simulink model "gm_sampleModel71194_pp_7_1_sub"  (R2023b)
settings: Solver=VariableStepAuto  StartTime=0.0  StopTime=10.0  RelTol=1e-3
libraries: simulink x45, hdlsllib x1, hdlmdlgenlib x1
(part 1 of 2)
settings Model: Creator=CW  LastModifiedBy=CW
settings OptimizationCC: BlockReduction=off  ConditionallyExecuteInputs=off
settings DebuggingCC: ArtificialAlgebraicLoopMsg=none  InheritedTsInSrcMsg=none

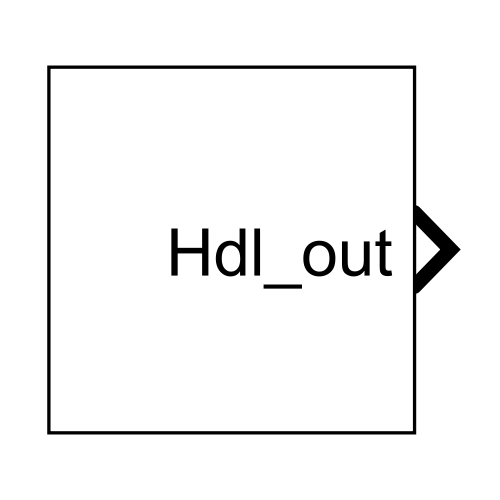
[thumbnail: Simulink's stored preview of the top-level diagram]
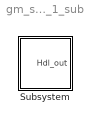
== system gm_sampleModel71194_pp_7_1_sub ==
  Subsystem : Subsystem

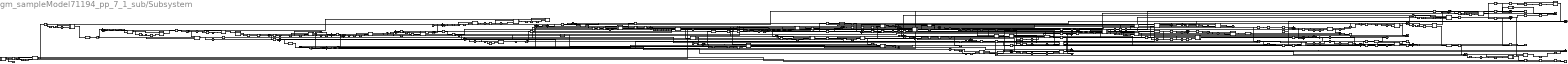
== system gm_sampleModel71194_pp_7_1_sub/Subsystem ==
  Reshape : Reshape
  Reshape1 : Reshape
  cfblk1 : Subsystem
  cfblk10 : Subsystem  mask(Compare To Zero){relop=<=, OutDataTypeStr=uint8, ZeroCross=on}
      mask prompts: relop "Simulink:masks:Operator_MP"; OutDataTypeStr "Simulink:masks:OutputDataType_MP"; ZeroCross "Simulink:masks:EnableZerocrossingDetection_MP"
      mask help: Simulink:masks:CompareToZero_MD
      mask init:
      | OutDataTypeStr = 'uint8';
      | ZeroCross = 'on';
      | blkName = 'sampleModel71194_pp_7_1_sub/Subsystem/cfblk10';
      | relop = '<=';
      | setValue = 'fixdt(0, 8)';
      mask TypeOptions relop: == | ~= | < | <= | >= | >
      mask TypeOptions OutDataTypeStr: Simulink:masks:uint8 | Simulink:masks:boolean
      mask Callback ZeroCross: sl('zeroCrossEnable', gcbh);
      mask Display: disp([relop,' 0'])
  cfblk100_inst : Subsystem
  cfblk{18,21,41,43,80..82,92,101,118,121,123} (12 alike) : Product  Inputs=*/  OutDataTypeStr=uint8  RndMeth=Zero  SaturateOnIntegerOverflow=on  SampleTime=1
  cfblk102_inst : Subsystem
  cfblk103 : Subsystem
  cfblk{20,22,29,33,36,40,64,72,77,88,90,94,104,111..112,115..116,125,128,141,143..144,152} (23 alike) : Sum  OutDataTypeStr=uint8  AccumDataTypeStr=uint8  SampleTime=1
  cfblk{49,58..59,74,105,108,110} (7 alike) : Signum  SampleTime=1
  cfblk{15,32,35,48,61,85,106,113,139..140} (10 alike) : MinMax  OutDataTypeStr=uint8
  cfblk{16,70,89,91,99,109,120,137,142,151} (10 alike) : Sum  Inputs=+-  OutDataTypeStr=uint8  AccumDataTypeStr=uint8  SampleTime=1
  cfblk11 : Subsystem
  cfblk{56,73,97,114,122} (5 alike) : ComplexToRealImag  SampleTime=1
  cfblk{34,53,69,71,86,96,98,117} (8 alike) : Sum  OutDataTypeStr=uint8  AccumDataTypeStr=uint8  RndMeth=Nearest  SampleTime=1
  cfblk117_const_val : Constant  Value=0  VectorParams1D=off  OutDataTypeStr=uint8  SampleTime=1
  cfblk119_inst : Subsystem
  cfblk12 : simulink/Logic and Bit Operations/Bit Set  iBit=double(0)
  cfblk124 : Subsystem  mask(Real World Value Increment){}
      mask help: Simulink:masks:RealWorldValueIncrement_MD
      mask Display: disp('V++')
  cfblk126_inst : Subsystem
  cfblk127 : Subsystem
  cfblk129 : Subsystem  mask(Real World Value Increment){}
      mask help: Simulink:masks:RealWorldValueIncrement_MD
      mask Display: disp('V++')
  cfblk13 : Subsystem  mask(Compare To Constant){relop=<=, const=double(3), OutDataTypeStr=uint8, ZeroCross=on}
      mask prompts: relop "Simulink:masks:Operator_MP"; const "Simulink:masks:ConstantValue_MP"; OutDataTypeStr "Simulink:masks:OutputDataType_MP"; ZeroCross "Simulink:masks:EnableZerocrossingDetection_MP"
      mask help: Simulink:masks:CompareToConstant_MD
      mask init:
      | OutDataTypeStr = 'uint8';
      | ZeroCross = 'on';
      | blkName = 'sampleModel71194_pp_7_1_sub/Subsystem/cfblk13';
      | const = double(3);
      | const_str = '3.0';
      | const_val = double(3);
      | relop = '<=';
      | setValue = 'fixdt(0, 8)';
      | str = '<= 3';
      mask TypeOptions relop: == | ~= | < | <= | >= | >
      mask TypeOptions OutDataTypeStr: Simulink:masks:uint8 | Simulink:masks:boolean
      mask Callback ZeroCross: sl('zeroCrossEnable', gcbh);
      mask Display: disp(str)
  cfblk130 : Subsystem
  cfblk131 : Subsystem
  cfblk{26,44,51,62,132,148} (6 alike) : Abs  SampleTime=1  OutDataTypeStr=uint8  SaturateOnIntegerOverflow=off
  cfblk133 : Subsystem
  cfblk134_inst : Subsystem
  cfblk135 : Subsystem
  cfblk136 : Subsystem
  cfblk{42,57,66,68,78..79,138,145..146} (9 alike) : Sum  Inputs=+  OutDataTypeStr=uint8
  cfblk14 : Subsystem  mask(Detect Fall Nonpositive){vinit=double(0), InputProcessing=Elements as channels (sample based), OutDataTypeStr=uint8}
      mask prompts: vinit "Simulink:masks:InitialCondition_MP"; InputProcessing "Simulink:masks:InputProcessing_MP"; OutDataTypeStr "Simulink:masks:OutputDataType_MP"
      mask help: Simulink:masks:DetectFallNonpositive_MD
      mask init:
      | InputProcessing = 'Elements as channels (sample based)';
      | OutDataTypeStr = 'uint8';
      | vinit = double(0);
      mask TypeOptions InputProcessing: Simulink:masks:ColumnsAsChannelsFrameBased | Simulink:masks:ElementsAsChannelsSampleBased
      mask TypeOptions OutDataTypeStr: Simulink:masks:uint8 | Simulink:masks:boolean
      mask Display: fprintf('U <= 0\n&  NOT\nU/z <= 0')
  cfblk147 : Subsystem
  cfblk149 : Sum  OutDataTypeStr=uint8  AccumDataTypeStr=uint32  SampleTime=1
  cfblk150 : Subsystem
  cfblk153 : Subsystem
  cfblk156 : Constant  OutDataTypeStr=uint8  SampleTime=1
  cfblk157 : Constant  OutDataTypeStr=uint8  SampleTime=1
  cfblk158 : hdlsllib/Sources/HDL Counter  CountType=Count limited  CountInit=0  CountStep=1  CountMax=25  CountFromType=Initial value  CountFrom=0  CountResetPort=off  CountLoadPort=off  CountEnbPort=off  CountDirPort=off  CountHitOutputPort=off  CountDataType=Unsigned  CountWordLen=8  CountFracLen=0  CountSampTime=1
  cfblk159 : Constant  Value=0  VectorParams1D=off  OutDataTypeStr=uint8  SampleTime=1
  cfblk160 : Subsystem
  cfblk161 : Subsystem
  cfblk162 : Subsystem
  cfblk{163..170} (8 alike) : Switch  Threshold=double(0)  OutDataTypeStr=uint8  SampleTime=1  SaturateOnIntegerOverflow=off  InputSameDT=off
  cfblk17 : Subsystem
  cfblk{171..173,175..200} (29 alike) : Delay  DelayLength=double(2)  InitialCondition=0  SampleTime=1
  cfblk174 : Subsystem
  cfblk19 : Subsystem
  cfblk2 : Subsystem
  cfblk{201..203,205,207..208,215,218..219} (9 alike) : DataTypeConversion  OutDataTypeStr=fixdt(0,8,0)
  cfblk204 : Subsystem
  cfblk206 : Subsystem
  cfblk209 : Subsystem
  cfblk210 : DataTypeConversion  OutDataTypeStr=uint8  SampleTime=1  SaturateOnIntegerOverflow=off  RndMeth=Floor
  cfblk211 : Subsystem
  cfblk212 : DataTypeConversion  OutDataTypeStr=uint8  SampleTime=1  SaturateOnIntegerOverflow=off  RndMeth=Floor
  cfblk213 : Subsystem
  cfblk214 : Subsystem
  cfblk216 : Subsystem
  cfblk217 : Subsystem
  cfblk220 : Subsystem
  cfblk23 : Subsystem
  cfblk{24,76,83..84} (4 alike) : Gain  Gain="fi(0,0,8,7,\"hex\",\"80\")"  ParamDataTypeStr=fixdt(0, 8, 7)  OutDataTypeStr=uint8  SampleTime=1
  cfblk27 : Subsystem
  cfblk3 : RelationalOperator  Operator=<=  OutDataTypeStr=fixdt(0,8,0)  SampleTime=1  InputSameDT=off
  cfblk30 : Subsystem
  cfblk31_inst : Subsystem
  cfblk34_const_val : Constant  Value=0  VectorParams1D=off  OutDataTypeStr=uint8  SampleTime=1
  cfblk37 : Subsystem
  cfblk38 : Subsystem  mask(Real World Value Increment){}
      mask help: Simulink:masks:RealWorldValueIncrement_MD
      mask Display: disp('V++')
  cfblk39 : Subsystem
  cfblk4 : Logic  AllPortsSameDT=off  OutDataTypeStr=boolean  SampleTime=1
  cfblk45 : Subsystem
  cfblk46 : Subsystem
  cfblk5 : hdlmdlgenlib/Buffer
  cfblk50 : Subsystem
  cfblk52 : Subsystem  mask(Real World Value Increment){}
      mask help: Simulink:masks:RealWorldValueIncrement_MD
      mask Display: disp('V++')
  cfblk53_const_val : Constant  Value=0  VectorParams1D=off  OutDataTypeStr=uint8  SampleTime=1
  cfblk54 : Subsystem
  cfblk55 : Subsystem  mask(Real World Value Increment){}
      mask help: Simulink:masks:RealWorldValueIncrement_MD
      mask Display: disp('V++')
  cfblk6 : Subsystem
  cfblk60 : Subsystem  mask(Real World Value Increment){}
      mask help: Simulink:masks:RealWorldValueIncrement_MD
      mask Display: disp('V++')
  cfblk63 : Subsystem
  cfblk65 : Subsystem
  cfblk67 : Subsystem
  cfblk69_const_val : Constant  Value=0  VectorParams1D=off  OutDataTypeStr=uint8  SampleTime=1
  cfblk7 : Subsystem  mask(Compare To Zero){relop=<=, OutDataTypeStr=uint8, ZeroCross=on}
      mask prompts: relop "Simulink:masks:Operator_MP"; OutDataTypeStr "Simulink:masks:OutputDataType_MP"; ZeroCross "Simulink:masks:EnableZerocrossingDetection_MP"
      mask help: Simulink:masks:CompareToZero_MD
      mask init:
      | OutDataTypeStr = 'uint8';
      | ZeroCross = 'on';
      | blkName = 'sampleModel71194_pp_7_1_sub/Subsystem/cfblk7';
      | relop = '<=';
      | setValue = 'fixdt(0, 8)';
      mask TypeOptions relop: == | ~= | < | <= | >= | >
      mask TypeOptions OutDataTypeStr: Simulink:masks:uint8 | Simulink:masks:boolean
      mask Callback ZeroCross: sl('zeroCrossEnable', gcbh);
      mask Display: disp([relop,' 0'])
  cfblk71_const_val : Constant  Value=0  VectorParams1D=off  OutDataTypeStr=uint8  SampleTime=1
  cfblk75 : Subsystem  mask(Real World Value Increment){}
      mask help: Simulink:masks:RealWorldValueIncrement_MD
      mask Display: disp('V++')
  cfblk8 : simulink/Logic and Bit Operations/Bitwise Operator  logicop=AND  UseBitMask=on  BitMask="fi(0,0,1,0,\"hex\",\"1\")"  BitMaskRealWorld=Real World Value
  cfblk86_const_val : Constant  Value=0  VectorParams1D=off  OutDataTypeStr=uint8  SampleTime=1
  cfblk87_inst : Subsystem
  cfblk9 : simulink/Logic and Bit Operations/Detect Increase  vinit=0.0  OutDataTypeStr=uint8
      settings: LibrarySourceBlock=|
      | hdlsllib/Logic and Bit
      | Operations/Detect
      | Increase
  cfblk93 : Subsystem
  cfblk95 : Subsystem
  cfblk96_const_val : Constant  Value=0  VectorParams1D=off  OutDataTypeStr=uint8  SampleTime=1
  cfblk98_const_val : Constant  Value=0  VectorParams1D=off  OutDataTypeStr=uint8  SampleTime=1
  compare{,10,14,17,22,26,30,36} (8 alike) : simulink/Logic and Bit Operations/Compare To Constant  relop=>=  const=255  OutDataTypeStr=boolean
  compare{1,11..12,24..25,29,31..32,39} (9 alike) : simulink/Logic and Bit Operations/Compare To Constant  relop=>=  const=1  OutDataTypeStr=boolean
  compare{2..9,13,15..16,18..21,23,33..35,37..38} (21 alike) : simulink/Logic and Bit Operations/Compare To Constant  relop=>=  const=0  OutDataTypeStr=boolean
  compare27 : simulink/Logic and Bit Operations/Compare To Constant  relop=>=  const=2  OutDataTypeStr=boolean
  compare28 : simulink/Logic and Bit Operations/Compare To Constant  relop=>=  const=3  OutDataTypeStr=boolean
  emi_{6,14,22,31,39,48,56,64,72,80,88,96,104,112,121,129,137,145,153,161,169,177,193,209,218,227,235,243,251,260,268,276,284,300,308,316,325} (37 alike) : DataTypeConversion  OutDataTypeStr=fixdt(0,8,0)
  emi_{73,105,178,210,228,269,301,326} (8 alike) : Delay  DelayLength=double(2)  InitialCondition=255  SampleTime=1
  emi_{40,49,97,113,186,194,285,293,317} (9 alike) : Delay  DelayLength=double(2)  InitialCondition=1  SampleTime=1
  emi_{7,15,23,57,65,81,89,122,130,138,146,154,162,170,202,219,236,244,252,261,277} (21 alike) : Delay  DelayLength=double(2)  InitialCondition=0  SampleTime=1
  emi_185 : DataTypeConversion  OutDataTypeStr=uint8  SampleTime=1  SaturateOnIntegerOverflow=off  RndMeth=Floor
  emi_201 : DataTypeConversion  OutDataTypeStr=uint8  SampleTime=1  SaturateOnIntegerOverflow=off  RndMeth=Floor
  emi_292 : DataTypeConversion  OutDataTypeStr=uint8  SampleTime=1  SaturateOnIntegerOverflow=off  RndMeth=Floor
  emi_309 : Delay  DelayLength=double(2)  InitialCondition=3  SampleTime=1
  emi_32 : Delay  DelayLength=double(2)  InitialCondition=2  SampleTime=1
  Hdl_out : Outport  OutDataTypeStr=uint8  SampleTime=1
  wires:
  cfblk1/1(emi_2) -> emi_236/1, Hdl_out/1, cfblk220/1(emi_230)
  cfblk10/1(y) -> cfblk21/1
  cfblk100_inst/1(out1) -> emi_219/1, cfblk65/1(emi_212)
  cfblk101/1 -> cfblk138/1
  cfblk102_inst/1(out1) -> cfblk203/1
  cfblk103/1(emi_10) -> cfblk124/1(u)
  cfblk104/1 -> cfblk129/1(u)
  cfblk105/1 -> cfblk122/1
  cfblk106/1 -> cfblk134_inst/1(in1), cfblk172/1
  cfblk108/1 -> emi_317/1, cfblk95/1(emi_311)
  cfblk109/1 -> cfblk99/2, cfblk90/1
  cfblk11/1(emi_18) -> cfblk201/1
  cfblk110/1 -> cfblk112/2, cfblk57/1
  cfblk111/1 -> emi_40/1, cfblk130/1(emi_34)
  cfblk112/1 -> emi_269/1, cfblk46/1(emi_263)
  cfblk113/1 -> emi_130/1, cfblk2/1(emi_124), cfblk35/1
  cfblk114/1 -> cfblk110/1
  cfblk114/2 -> cfblk163/3
  cfblk115/1 -> emi_32/1, cfblk127/1(emi_25)
  cfblk116/1 -> cfblk18/1
  cfblk117/1 -> emi_178/1, cfblk213/1(emi_172)
  cfblk118/1 -> cfblk36/1
  cfblk119_inst/1(out1) -> cfblk196/1
  cfblk12/1 -> cfblk212/1
  cfblk120/1 -> emi_89/1, cfblk147/1(emi_83)
  cfblk121/1 -> cfblk85/1
  cfblk122/1 -> cfblk142/1
  cfblk122/2 -> cfblk15/1
  cfblk123/1 -> cfblk161/1(In1)
  cfblk124/1(y) -> cfblk34/1
  cfblk125/1 -> emi_97/1, cfblk150/1(emi_91)
  cfblk126_inst/1(out1) -> cfblk193/1, cfblk192/1
  cfblk127/1(emi_26) -> cfblk100_inst/2(in2)
  cfblk127/2(emi_27) -> cfblk91/2, cfblk164/2
  cfblk128/1 -> cfblk77/2, emi_252/1, cfblk39/1(emi_246)
  cfblk129/1(y) -> cfblk170/2
  cfblk13/1(y) -> cfblk32/1
  cfblk130/1(emi_35) -> cfblk52/1(u)
  cfblk131/1(emi_43) -> cfblk140/1
  cfblk131/2(emi_44) -> cfblk164/3
  cfblk132/1 -> cfblk167/2, emi_73/1, cfblk136/1(emi_67)
  cfblk133/1(emi_52) -> cfblk190/1
  cfblk134_inst/1(out1) -> cfblk40/2
  cfblk135/1(emi_60) -> emi_202/1, cfblk217/1(emi_196)
  cfblk136/1(emi_68) -> cfblk137/1
  cfblk137/1 -> cfblk33/2, cfblk123/2
  cfblk138/1 -> cfblk38/1(u)
  cfblk139/1 -> cfblk215/1
  cfblk14/1(Y) -> Reshape/1
  cfblk140/1 -> cfblk164/1
  cfblk141/1 -> cfblk114/1
  cfblk142/1 -> cfblk76/1
  cfblk143/1 -> emi_105/1, cfblk153/1(emi_99)
  cfblk144/1 -> emi_154/1, cfblk209/1(emi_148), cfblk60/1(u)
  cfblk145/1 -> cfblk119_inst/2(in2), cfblk83/1
  cfblk146/1 -> cfblk183/1
  cfblk147/1(emi_84) -> cfblk31_inst/2(in2), cfblk205/1
  cfblk148/1 -> cfblk36/2
  cfblk149/1 -> cfblk116/1
  cfblk15/1 -> cfblk137/2, cfblk101/2
  cfblk150/1(emi_92) -> emi_194/1, cfblk216/1(emi_188)
  cfblk151/1 -> emi_81/1, cfblk174/1(emi_75)
  cfblk152/1 -> emi_277/1, cfblk13/1(u), cfblk50/1(emi_271)
  cfblk153/1(emi_100) -> cfblk24/1
  cfblk156/1 -> cfblk91/1
  cfblk157/1 -> cfblk89/2, cfblk72/1
  cfblk158/1 -> cfblk152/1
  cfblk159/1 -> cfblk166/3
  cfblk16/1 -> cfblk144/1
  cfblk160/1(Out1) -> cfblk109/2
  cfblk161/1(Out1) -> cfblk188/1
  cfblk162/1(Out1) -> cfblk175/1
  cfblk163/1 -> cfblk166/2
  cfblk164/1 -> emi_285/1, cfblk54/1(emi_279)
  cfblk165/1 -> cfblk187/1
  cfblk166/1 -> cfblk185/1
  cfblk167/1 -> cfblk189/1
  cfblk168/1 -> cfblk20/1
  cfblk169/1 -> emi_162/1, cfblk211/1(emi_156)
  cfblk17/1(emi_108) -> cfblk165/1, cfblk80/1
  cfblk170/1 -> cfblk43/1
  cfblk171/1 -> cfblk18/2
  cfblk172/1 -> cfblk120/1
  cfblk173/1 -> cfblk116/2
  cfblk174/1(emi_76) -> cfblk219/1
  cfblk175/1 -> cfblk169/2
  cfblk176/1 -> cfblk16/2
  cfblk177/1 -> cfblk170/1
  cfblk178/1 -> cfblk111/2
  cfblk179/1 -> cfblk141/2
  cfblk18/1 -> cfblk33/1
  cfblk180/1 -> cfblk100_inst/1(in1)
  cfblk181/1 -> cfblk20/2
  cfblk182/1 -> cfblk208/1
  cfblk183/1 -> cfblk70/2
  cfblk184/1 -> cfblk88/1
  cfblk185/1 -> cfblk109/1
  cfblk186/1 -> cfblk92/2
  cfblk187/1 -> cfblk41/1
  cfblk188/1 -> cfblk94/1
  cfblk189/1 -> cfblk99/1
  cfblk19/1(emi_117) -> cfblk49/1, cfblk165/2
  cfblk190/1 -> cfblk81/1
  cfblk191/1 -> cfblk144/2
  cfblk192/1 -> cfblk128/1
  cfblk193/1 -> cfblk168/3
  cfblk194/1 -> cfblk112/1
  cfblk195/1 -> cfblk104/2
  cfblk196/1 -> cfblk168/1
  cfblk197/1 -> cfblk82/2
  cfblk198/1 -> cfblk43/2
  cfblk199/1 -> cfblk170/3
  cfblk2/1(emi_125) -> cfblk3/1
  cfblk20/1 -> cfblk16/1
  cfblk200/1 -> cfblk31_inst/1(in1)
  cfblk201/1 -> cfblk148/1
  cfblk202/1 -> emi_23/1, cfblk11/1(emi_17)
  cfblk203/1 -> cfblk145/1
  cfblk204/1(emi_133) -> cfblk102_inst/1(in1)
  cfblk205/1 -> cfblk102_inst/2(in2)
  cfblk206/1(emi_141) -> emi_170/1, emi_122/1, cfblk27/1(emi_164), cfblk19/1(emi_115)
  cfblk207/1 -> cfblk29/1
  cfblk208/1 -> cfblk29/2
  cfblk209/1(emi_149) -> cfblk8/1
  cfblk21/1 -> emi_326/1, cfblk93/1(emi_319)
  cfblk210/1 -> cfblk4/1, cfblk151/2
  cfblk211/1(emi_157) -> cfblk12/1
  cfblk212/1 -> cfblk42/1
  cfblk213/1(emi_173) -> emi_293/1, cfblk6/1(emi_287)
  cfblk214/1(emi_181) -> cfblk125/2
  cfblk215/1 -> cfblk126_inst/1(in1), emi_138/1, cfblk204/1(emi_132)
  cfblk216/1(emi_189) -> cfblk139/1
  cfblk217/1(emi_197) -> cfblk86/1, cfblk51/1
  cfblk218/1 -> emi_65/1, cfblk135/1(emi_59)
  cfblk219/1 -> emi_7/1, cfblk1/1(emi_1)
  cfblk22/1 -> emi_228/1, cfblk30/1(emi_221), cfblk81/2
  cfblk220/1(emi_231) -> cfblk58/1, cfblk80/2
  cfblk23/1(emi_205) -> cfblk89/1, cfblk22/2
  cfblk24/1 -> cfblk117/1, cfblk61/1
  Reshape/1 -> cfblk151/1
  cfblk26/1 -> Reshape1/1
  cfblk27/1(emi_165) -> cfblk149/2
  cfblk29/1 -> emi_146/1, cfblk206/1(emi_140)
  cfblk3/1 -> cfblk177/1
  cfblk30/1(emi_222) -> cfblk69/1
  cfblk30/2(emi_223) -> cfblk14/1(U)
  cfblk31_inst/1(out1) -> cfblk152/2
  cfblk32/1 -> cfblk163/2
  cfblk33/1 -> cfblk10/1(u)
  cfblk34/1 -> cfblk78/1
  cfblk35/1 -> cfblk178/1
  cfblk36/1 -> cfblk194/1
  cfblk37/1(emi_239) -> cfblk9/1
  cfblk38/1(y) -> cfblk182/1, cfblk181/1
  cfblk39/1(emi_247) -> cfblk184/1
  cfblk4/1 -> cfblk149/1
  cfblk40/1 -> cfblk108/1
  cfblk41/1 -> emi_15/1, cfblk103/1(emi_9)
  cfblk42/1 -> cfblk44/1
  cfblk43/1 -> cfblk73/1, cfblk118/2
  cfblk44/1 -> cfblk55/1(u)
  cfblk45/1(emi_255) -> cfblk56/1
  cfblk45/2(emi_256) -> cfblk163/1
  cfblk46/1(emi_264) -> cfblk75/1(u)
  Reshape1/1 -> cfblk59/1
  cfblk48/1 -> cfblk128/2
  cfblk49/1 -> cfblk134_inst/2(in2), cfblk115/2, cfblk160/1(In1), cfblk113/1
  cfblk5/1 -> cfblk90/2, cfblk3/2
  cfblk50/1(emi_272) -> cfblk168/2
  cfblk51/1 -> cfblk119_inst/1(in1), cfblk21/2
  cfblk52/1(y) -> cfblk169/1, cfblk121/2
  cfblk53/1 -> cfblk180/1
  cfblk54/1(emi_280) -> cfblk87_inst/1(in1)
  cfblk55/1(y) -> cfblk64/1
  cfblk56/1 -> cfblk48/1
  cfblk56/2 -> cfblk4/2, cfblk123/1
  cfblk57/1 -> emi_49/1, cfblk131/1(emi_42)
  cfblk58/1 -> emi_244/1, cfblk37/1(emi_238), cfblk68/1
  cfblk59/1 -> cfblk199/1, cfblk198/1, cfblk92/1
  cfblk6/1(emi_288) -> emi_186/1, cfblk214/1(emi_180)
  cfblk60/1(y) -> cfblk88/2
  cfblk61/1 -> cfblk74/1
  cfblk62/1 -> cfblk162/1(In1)
  cfblk63/1(emi_296) -> cfblk5/1, cfblk132/1
  cfblk64/1 -> cfblk62/1, emi_309/1, cfblk67/1(emi_303)
  cfblk65/1(emi_213) -> cfblk179/1
  cfblk65/2(emi_214) -> cfblk53/1
  cfblk66/1 -> cfblk176/1
  cfblk67/1(emi_304) -> cfblk97/1
  cfblk68/1 -> cfblk167/3, cfblk7/1(u)
  cfblk69/1 -> emi_301/1, cfblk63/1(emi_295)
  cfblk7/1(y) -> cfblk70/1
  cfblk70/1 -> cfblk120/2
  cfblk71/1 -> cfblk72/2, cfblk22/1, emi_113/1, cfblk17/1(emi_107)
  cfblk72/1 -> cfblk142/2
  cfblk73/1 -> cfblk141/1
  cfblk73/2 -> cfblk167/1
  cfblk74/1 -> cfblk165/3, cfblk191/1
  cfblk75/1(y) -> cfblk207/1, cfblk143/2
  cfblk76/1 -> cfblk197/1
  cfblk77/1 -> cfblk26/1
  cfblk78/1 -> cfblk115/1, cfblk121/1
  cfblk79/1 -> cfblk71/1
  cfblk8/1 -> cfblk210/1
  cfblk80/1 -> cfblk186/1
  cfblk81/1 -> cfblk143/1, emi_57/1, cfblk133/1(emi_51)
  cfblk82/1 -> cfblk166/1, cfblk41/2
  cfblk83/1 -> cfblk202/1, cfblk195/1, cfblk118/1
  cfblk84/1 -> cfblk126_inst/2(in2), cfblk125/1
  cfblk85/1 -> cfblk79/1
  cfblk86/1 -> cfblk105/1
  cfblk87_inst/1(out1) -> cfblk66/1
  cfblk88/1 -> cfblk98/1, cfblk40/1
  cfblk89/1 -> cfblk94/2
  cfblk9/1 -> cfblk169/3, cfblk84/1
  cfblk90/1 -> cfblk87_inst/2(in2), cfblk146/1
  cfblk91/1 -> cfblk101/1
  cfblk92/1 -> emi_210/1, cfblk23/1(emi_204)
  cfblk93/1(emi_320) -> cfblk171/1
  cfblk93/2(emi_321) -> cfblk106/1
  cfblk94/1 -> cfblk82/1
  cfblk95/1(emi_312) -> cfblk173/1
  cfblk96/1 -> cfblk200/1
  cfblk97/1 -> cfblk104/1
  cfblk97/2 -> cfblk96/1
  cfblk98/1 -> cfblk77/1, cfblk64/2, cfblk111/1
  cfblk99/1 -> cfblk218/1, emi_261/1, cfblk45/1(emi_254)
  emi_104/1 -> compare/1
  emi_105/1 -> emi_104/1
  emi_112/1 -> compare1/1
  emi_113/1 -> emi_112/1
  emi_121/1 -> compare2/1
  emi_122/1 -> emi_121/1
  emi_129/1 -> compare3/1
  emi_130/1 -> emi_129/1
  emi_137/1 -> compare5/1
  emi_138/1 -> emi_137/1
  emi_14/1 -> compare4/1
  emi_145/1 -> compare6/1
  emi_146/1 -> emi_145/1
  emi_15/1 -> emi_14/1
  emi_153/1 -> compare7/1
  emi_154/1 -> emi_153/1
  emi_161/1 -> compare8/1
  emi_162/1 -> emi_161/1
  emi_169/1 -> compare9/1
  emi_170/1 -> emi_169/1
  emi_177/1 -> compare10/1
  emi_178/1 -> emi_177/1
  emi_185/1 -> compare11/1
  emi_186/1 -> emi_185/1
  emi_193/1 -> compare12/1
  emi_194/1 -> emi_193/1
  emi_201/1 -> compare13/1
  emi_202/1 -> emi_201/1
  emi_209/1 -> compare14/1
  emi_210/1 -> emi_209/1
  emi_218/1 -> compare16/1
  emi_219/1 -> emi_218/1
  emi_22/1 -> compare15/1
  emi_227/1 -> compare17/1
  emi_228/1 -> emi_227/1
  emi_23/1 -> emi_22/1
  emi_235/1 -> compare18/1
  emi_236/1 -> emi_235/1
  emi_243/1 -> compare19/1
  emi_244/1 -> emi_243/1
  emi_251/1 -> compare20/1
  emi_252/1 -> emi_251/1
  emi_260/1 -> compare21/1
  emi_261/1 -> emi_260/1
  emi_268/1 -> compare22/1
  emi_269/1 -> emi_268/1
  emi_276/1 -> compare23/1
  emi_277/1 -> emi_276/1
  emi_284/1 -> compare24/1
  emi_285/1 -> emi_284/1
  emi_292/1 -> compare25/1
  emi_293/1 -> emi_292/1
  emi_300/1 -> compare26/1
  emi_301/1 -> emi_300/1
  emi_308/1 -> compare28/1
  emi_309/1 -> emi_308/1
  emi_31/1 -> compare27/1
  emi_316/1 -> compare29/1
  emi_317/1 -> emi_316/1
  emi_32/1 -> emi_31/1
  emi_325/1 -> compare30/1
  emi_326/1 -> emi_325/1
  emi_39/1 -> compare31/1
  emi_40/1 -> emi_39/1
  emi_48/1 -> compare32/1
  emi_49/1 -> emi_48/1
  emi_56/1 -> compare34/1
  emi_57/1 -> emi_56/1
  emi_6/1 -> compare33/1
  emi_64/1 -> compare35/1
  emi_65/1 -> emi_64/1
  emi_7/1 -> emi_6/1
  emi_72/1 -> compare36/1
  emi_73/1 -> emi_72/1
  emi_80/1 -> compare37/1
  emi_81/1 -> emi_80/1
  emi_88/1 -> compare38/1
  emi_89/1 -> emi_88/1
  emi_96/1 -> compare39/1
  emi_97/1 -> emi_96/1
  cfblk117_const_val/1 -> cfblk117/2
  cfblk34_const_val/1 -> cfblk34/2
  cfblk53_const_val/1 -> cfblk53/2
  cfblk69_const_val/1 -> cfblk69/2
  cfblk71_const_val/1 -> cfblk71/2
  cfblk86_const_val/1 -> cfblk86/2
  cfblk96_const_val/1 -> cfblk96/2
  cfblk98_const_val/1 -> cfblk98/2
  compare/1 -> cfblk153/2(Action Port)
  compare1/1 -> cfblk17/2(Action Port)
  compare2/1 -> cfblk19/2(Action Port)
  compare3/1 -> cfblk2/2(Action Port)
  compare4/1 -> cfblk103/2(Action Port)
  compare5/1 -> cfblk204/2(Action Port)
  compare6/1 -> cfblk206/2(Action Port)
  compare7/1 -> cfblk209/2(Action Port)
  compare8/1 -> cfblk211/2(Action Port)
  compare9/1 -> cfblk27/2(Action Port)
  compare10/1 -> cfblk213/2(Action Port)
  compare11/1 -> cfblk214/2(Action Port)
  compare12/1 -> cfblk216/2(Action Port)
  compare13/1 -> cfblk217/2(Action Port)
  compare14/1 -> cfblk23/2(Action Port)
  compare15/1 -> cfblk11/2(Action Port)
  compare16/1 -> cfblk65/2(Action Port)
  compare17/1 -> cfblk30/2(Action Port)
  compare18/1 -> cfblk220/2(Action Port)
  compare19/1 -> cfblk37/2(Action Port)
  compare20/1 -> cfblk39/2(Action Port)
  compare21/1 -> cfblk45/2(Action Port)
  compare22/1 -> cfblk46/2(Action Port)
  compare23/1 -> cfblk50/2(Action Port)
  compare24/1 -> cfblk54/2(Action Port)
  compare25/1 -> cfblk6/2(Action Port)
  compare26/1 -> cfblk63/2(Action Port)
  compare27/1 -> cfblk127/2(Action Port)
  compare28/1 -> cfblk67/2(Action Port)
  compare29/1 -> cfblk95/2(Action Port)
  compare30/1 -> cfblk93/2(Action Port)
  compare31/1 -> cfblk130/2(Action Port)
  compare32/1 -> cfblk131/2(Action Port)
  compare33/1 -> cfblk1/2(Action Port)
  compare34/1 -> cfblk133/2(Action Port)
  compare35/1 -> cfblk135/2(Action Port)
  compare36/1 -> cfblk136/2(Action Port)
  compare37/1 -> cfblk174/2(Action Port)
  compare38/1 -> cfblk147/2(Action Port)
  compare39/1 -> cfblk150/2(Action Port)

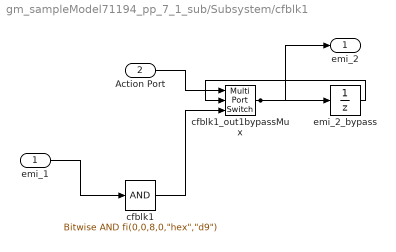
== system gm_sampleModel71194_pp_7_1_sub/Subsystem/cfblk1 ==
  emi_1 : Inport  OutDataTypeStr=uint8  PortDimensions=1  SampleTime=1
  Action Port : Inport  Port=2  OutDataTypeStr=boolean  SampleTime=1
  cfblk1 : simulink/Logic and Bit Operations/Bitwise Operator  logicop=AND  UseBitMask=on  BitMask="fi(0,0,8,0,\"hex\",\"d9\")"  BitMaskRealWorld=Real World Value
  cfblk1_out1bypassMux : MultiPortSwitch  DataPortOrder=Zero-based contiguous  Inputs=2  zeroidx=on  OutDataTypeStr=uint8  SampleTime=1  SaturateOnIntegerOverflow=off  InputSameDT=off
  emi_2_bypass : UnitDelay  InitialCondition="fi(0,0,8,0,\"hex\",\"00\")"  SampleTime=1
  emi_2 : Outport  SampleTime=1  InitialOutput=0
  wires:
  Action Port/1 -> cfblk1_out1bypassMux/1
  emi_1/1 -> cfblk1/1
  cfblk1/1 -> cfblk1_out1bypassMux/3
  cfblk1_out1bypassMux/1 -> emi_2_bypass/1, emi_2/1
  emi_2_bypass/1 -> cfblk1_out1bypassMux/2

== system gm_sampleModel71194_pp_7_1_sub/Subsystem/cfblk10 ==
  u : Inport  OutDataTypeStr=uint8  SampleTime=1
  Compare : RelationalOperator  Operator=<=  OutDataTypeStr=fixdt(0, 8)
  Constant : Constant  DisableCoverage=on  Value=0  OutDataTypeStr=Inherit: Inherit via back propagation  SampleTime=-1  PreserveConstantTs=on
  y : Outport  SampleTime=1
  wires:
  u/1 -> Compare/1
  Compare/1 -> y/1
  Constant/1 -> Compare/2

== system gm_sampleModel71194_pp_7_1_sub/Subsystem/cfblk100_inst ==
  in1 : Inport  OutDataTypeStr=uint8  SampleTime=1
  in2 : Inport  Port=2  OutDataTypeStr=uint8  SampleTime=1
  mul_cfblk100_dotp_mulcomp : Product  Inputs=**  OutDataTypeStr=uint8  SampleTime=1
  out1 : Outport  OutDataTypeStr=uint8  SampleTime=1
  wires:
  in1/1 -> mul_cfblk100_dotp_mulcomp/1
  in2/1 -> mul_cfblk100_dotp_mulcomp/2
  mul_cfblk100_dotp_mulcomp/1 -> out1/1

== system gm_sampleModel71194_pp_7_1_sub/Subsystem/cfblk102_inst ==
  in1 : Inport  OutDataTypeStr=uint8  SampleTime=1
  in2 : Inport  Port=2  OutDataTypeStr=uint8  SampleTime=1
  mul_cfblk102_dotp_mulcomp : Product  Inputs=**  OutDataTypeStr=uint8  SampleTime=1
  out1 : Outport  OutDataTypeStr=uint8  SampleTime=1
  wires:
  in1/1 -> mul_cfblk102_dotp_mulcomp/1
  in2/1 -> mul_cfblk102_dotp_mulcomp/2
  mul_cfblk102_dotp_mulcomp/1 -> out1/1

== system gm_sampleModel71194_pp_7_1_sub/Subsystem/cfblk103 ==
  emi_9 : Inport  OutDataTypeStr=uint8  PortDimensions=1  SampleTime=1
  Action Port : Inport  Port=2  OutDataTypeStr=boolean  SampleTime=1
  cfblk103 : Subsystem  mask(Real World Value Increment){}
      mask help: Simulink:masks:RealWorldValueIncrement_MD
      mask Display: disp('V++')
  cfblk103_out1bypassMux : MultiPortSwitch  DataPortOrder=Zero-based contiguous  Inputs=2  zeroidx=on  OutDataTypeStr=uint8  SampleTime=1  SaturateOnIntegerOverflow=off  InputSameDT=off
  emi_10_bypass : UnitDelay  InitialCondition="fi(0,0,8,0,\"hex\",\"00\")"  SampleTime=1
  emi_10 : Outport  SampleTime=1  InitialOutput=0
  wires:
  Action Port/1 -> cfblk103_out1bypassMux/1
  emi_9/1 -> cfblk103/1(u)
  cfblk103/1(y) -> cfblk103_out1bypassMux/3
  cfblk103_out1bypassMux/1 -> emi_10_bypass/1, emi_10/1
  emi_10_bypass/1 -> cfblk103_out1bypassMux/2

== system gm_sampleModel71194_pp_7_1_sub/Subsystem/cfblk11 ==
  emi_17 : Inport  OutDataTypeStr=uint8  PortDimensions=1  SampleTime=1
  Action Port : Inport  Port=2  OutDataTypeStr=boolean  SampleTime=1
  cfblk11 : Subsystem  mask(Detect Decrease){vinit=double(0), InputProcessing=Elements as channels (sample based), OutDataTypeStr=uint8}
      mask prompts: vinit "Simulink:masks:InitialCondition_MP"; InputProcessing "Simulink:masks:InputProcessing_MP"; OutDataTypeStr "Simulink:masks:OutputDataType_MP"
      mask help: Simulink:masks:DetectDecrease_MD
      mask TypeOptions InputProcessing: Simulink:masks:ColumnsAsChannelsFrameBased | Simulink:masks:ElementsAsChannelsSampleBased
      mask TypeOptions OutDataTypeStr: Simulink:masks:uint8 | Simulink:masks:boolean
      mask Display: fprintf('U < U/z')
  cfblk11_out1bypassMux : MultiPortSwitch  DataPortOrder=Zero-based contiguous  Inputs=2  zeroidx=on  OutDataTypeStr=uint8  SampleTime=1  SaturateOnIntegerOverflow=off  InputSameDT=off
  emi_18_bypass : UnitDelay  InitialCondition="fi(0,0,8,0,\"hex\",\"00\")"  SampleTime=1
  emi_18 : Outport  SampleTime=1  InitialOutput=0
  wires:
  Action Port/1 -> cfblk11_out1bypassMux/1, cfblk11/2(Action Port_out2)
  emi_17/1 -> cfblk11/1(U)
  cfblk11/1(Y) -> cfblk11_out1bypassMux/3
  cfblk11_out1bypassMux/1 -> emi_18_bypass/1, emi_18/1
  emi_18_bypass/1 -> cfblk11_out1bypassMux/2

== system gm_sampleModel71194_pp_7_1_sub/Subsystem/cfblk119_inst ==
  in1 : Inport  OutDataTypeStr=uint8  SampleTime=1
  in2 : Inport  Port=2  OutDataTypeStr=uint8  SampleTime=1
  mul_cfblk119_dotp_mulcomp : Product  Inputs=**  OutDataTypeStr=uint8  SampleTime=1
  out1 : Outport  OutDataTypeStr=uint8  SampleTime=1
  wires:
  in1/1 -> mul_cfblk119_dotp_mulcomp/1
  in2/1 -> mul_cfblk119_dotp_mulcomp/2
  mul_cfblk119_dotp_mulcomp/1 -> out1/1

== system gm_sampleModel71194_pp_7_1_sub/Subsystem/cfblk124 ==
  u : Inport  OutDataTypeStr=uint8  SampleTime=1
  FixPt Constant : Constant  DisableCoverage=on  OutDataTypeStr=Inherit: Inherit via back propagation  SampleTime=-1
  FixPt Data Type Duplicate : DataTypeDuplicate  DisableCoverage=on  NumInputPorts=3
  FixPt Sum1 : Sum  OutDataTypeStr=Inherit: Inherit via back propagation  InputSameDT=on  LockScale=on
  y : Outport  SampleTime=1
  wires:
  u/1 -> FixPt Sum1/1, FixPt Data Type Duplicate/2
  FixPt Constant/1 -> FixPt Sum1/2, FixPt Data Type Duplicate/3
  FixPt Sum1/1 -> FixPt Data Type Duplicate/1, y/1

== system gm_sampleModel71194_pp_7_1_sub/Subsystem/cfblk126_inst ==
  in1 : Inport  OutDataTypeStr=uint8  SampleTime=1
  in2 : Inport  Port=2  OutDataTypeStr=uint8  SampleTime=1
  mul_cfblk126_dotp_mulcomp : Product  Inputs=**  OutDataTypeStr=uint8  SampleTime=1
  out1 : Outport  OutDataTypeStr=uint8  SampleTime=1
  wires:
  in1/1 -> mul_cfblk126_dotp_mulcomp/1
  in2/1 -> mul_cfblk126_dotp_mulcomp/2
  mul_cfblk126_dotp_mulcomp/1 -> out1/1

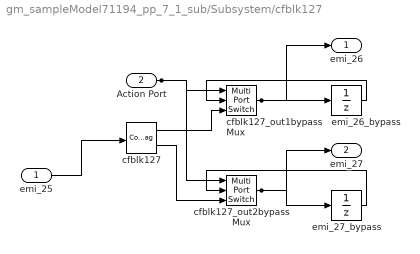
== system gm_sampleModel71194_pp_7_1_sub/Subsystem/cfblk127 ==
  emi_25 : Inport  OutDataTypeStr=uint8  PortDimensions=1  SampleTime=1
  Action Port : Inport  Port=2  OutDataTypeStr=boolean  SampleTime=1
  cfblk127 : ComplexToRealImag  SampleTime=1
  cfblk127_out1bypassMux : MultiPortSwitch  DataPortOrder=Zero-based contiguous  Inputs=2  zeroidx=on  OutDataTypeStr=uint8  SampleTime=1  SaturateOnIntegerOverflow=off  InputSameDT=off
  cfblk127_out2bypassMux : MultiPortSwitch  DataPortOrder=Zero-based contiguous  Inputs=2  zeroidx=on  OutDataTypeStr=uint8  SampleTime=1  SaturateOnIntegerOverflow=off  InputSameDT=off
  emi_26_bypass : UnitDelay  InitialCondition="fi(0,0,8,0,\"hex\",\"00\")"  SampleTime=1
  emi_27_bypass : UnitDelay  InitialCondition="fi(0,0,8,0,\"hex\",\"00\")"  SampleTime=1
  emi_26 : Outport  SampleTime=1  InitialOutput=0
  emi_27 : Outport  Port=2  SampleTime=1  InitialOutput=0
  wires:
  Action Port/1 -> cfblk127_out2bypassMux/1, cfblk127_out1bypassMux/1
  emi_25/1 -> cfblk127/1
  cfblk127/1 -> cfblk127_out1bypassMux/3
  cfblk127/2 -> cfblk127_out2bypassMux/3
  cfblk127_out1bypassMux/1 -> emi_26_bypass/1, emi_26/1
  emi_26_bypass/1 -> cfblk127_out1bypassMux/2
  cfblk127_out2bypassMux/1 -> emi_27_bypass/1, emi_27/1
  emi_27_bypass/1 -> cfblk127_out2bypassMux/2

== system gm_sampleModel71194_pp_7_1_sub/Subsystem/cfblk129 ==
  u : Inport  OutDataTypeStr=uint8  SampleTime=1
  FixPt Constant : Constant  DisableCoverage=on  OutDataTypeStr=Inherit: Inherit via back propagation  SampleTime=-1
  FixPt Data Type Duplicate : DataTypeDuplicate  DisableCoverage=on  NumInputPorts=3
  FixPt Sum1 : Sum  OutDataTypeStr=Inherit: Inherit via back propagation  InputSameDT=on  LockScale=on
  y : Outport  SampleTime=1
  wires:
  u/1 -> FixPt Sum1/1, FixPt Data Type Duplicate/2
  FixPt Constant/1 -> FixPt Sum1/2, FixPt Data Type Duplicate/3
  FixPt Sum1/1 -> FixPt Data Type Duplicate/1, y/1

== system gm_sampleModel71194_pp_7_1_sub/Subsystem/cfblk13 ==
  u : Inport  OutDataTypeStr=uint8  SampleTime=1
  Compare : RelationalOperator  Operator=<=  OutDataTypeStr=fixdt(0, 8)
  Constant : Constant  DisableCoverage=on  Value=const  OutDataTypeStr=Inherit: Inherit via back propagation  SampleTime=-1
  y : Outport  SampleTime=1
  wires:
  u/1 -> Compare/1
  Compare/1 -> y/1
  Constant/1 -> Compare/2

== system gm_sampleModel71194_pp_7_1_sub/Subsystem/cfblk130 ==
  emi_34 : Inport  OutDataTypeStr=uint8  PortDimensions=1  SampleTime=1
  Action Port : Inport  Port=2  OutDataTypeStr=boolean  SampleTime=1
  cfblk130 : Subsystem  mask(Real World Value Increment){}
      mask help: Simulink:masks:RealWorldValueIncrement_MD
      mask Display: disp('V++')
  cfblk130_out1bypassMux : MultiPortSwitch  DataPortOrder=Zero-based contiguous  Inputs=2  zeroidx=on  OutDataTypeStr=uint8  SampleTime=1  SaturateOnIntegerOverflow=off  InputSameDT=off
  emi_35_bypass : UnitDelay  InitialCondition="fi(0,0,8,0,\"hex\",\"00\")"  SampleTime=1
  emi_35 : Outport  SampleTime=1  InitialOutput=0
  wires:
  Action Port/1 -> cfblk130_out1bypassMux/1
  emi_34/1 -> cfblk130/1(u)
  cfblk130/1(y) -> cfblk130_out1bypassMux/3
  cfblk130_out1bypassMux/1 -> emi_35_bypass/1, emi_35/1
  emi_35_bypass/1 -> cfblk130_out1bypassMux/2

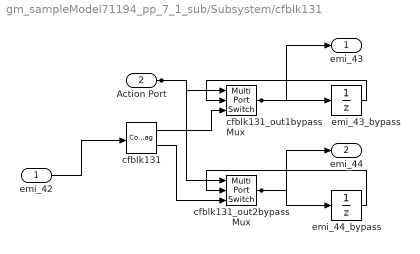
== system gm_sampleModel71194_pp_7_1_sub/Subsystem/cfblk131 ==
  emi_42 : Inport  OutDataTypeStr=uint8  PortDimensions=1  SampleTime=1
  Action Port : Inport  Port=2  OutDataTypeStr=boolean  SampleTime=1
  cfblk131 : ComplexToRealImag  SampleTime=1
  cfblk131_out1bypassMux : MultiPortSwitch  DataPortOrder=Zero-based contiguous  Inputs=2  zeroidx=on  OutDataTypeStr=uint8  SampleTime=1  SaturateOnIntegerOverflow=off  InputSameDT=off
  cfblk131_out2bypassMux : MultiPortSwitch  DataPortOrder=Zero-based contiguous  Inputs=2  zeroidx=on  OutDataTypeStr=uint8  SampleTime=1  SaturateOnIntegerOverflow=off  InputSameDT=off
  emi_43_bypass : UnitDelay  InitialCondition="fi(0,0,8,0,\"hex\",\"00\")"  SampleTime=1
  emi_44_bypass : UnitDelay  InitialCondition="fi(0,0,8,0,\"hex\",\"00\")"  SampleTime=1
  emi_43 : Outport  SampleTime=1  InitialOutput=0
  emi_44 : Outport  Port=2  SampleTime=1  InitialOutput=0
  wires:
  Action Port/1 -> cfblk131_out2bypassMux/1, cfblk131_out1bypassMux/1
  emi_42/1 -> cfblk131/1
  cfblk131/1 -> cfblk131_out1bypassMux/3
  cfblk131/2 -> cfblk131_out2bypassMux/3
  cfblk131_out1bypassMux/1 -> emi_43_bypass/1, emi_43/1
  emi_43_bypass/1 -> cfblk131_out1bypassMux/2
  cfblk131_out2bypassMux/1 -> emi_44_bypass/1, emi_44/1
  emi_44_bypass/1 -> cfblk131_out2bypassMux/2

== system gm_sampleModel71194_pp_7_1_sub/Subsystem/cfblk133 ==
  emi_51 : Inport  OutDataTypeStr=uint8  PortDimensions=1  SampleTime=1
  Action Port : Inport  Port=2  OutDataTypeStr=boolean  SampleTime=1
  cfblk133 : Signum  SampleTime=1
  cfblk133_out1bypassMux : MultiPortSwitch  DataPortOrder=Zero-based contiguous  Inputs=2  zeroidx=on  OutDataTypeStr=uint8  SampleTime=1  SaturateOnIntegerOverflow=off  InputSameDT=off
  emi_52_bypass : UnitDelay  InitialCondition="fi(0,0,8,0,\"hex\",\"00\")"  SampleTime=1
  emi_52 : Outport  SampleTime=1  InitialOutput=0
  wires:
  Action Port/1 -> cfblk133_out1bypassMux/1
  emi_51/1 -> cfblk133/1
  cfblk133/1 -> cfblk133_out1bypassMux/3
  cfblk133_out1bypassMux/1 -> emi_52_bypass/1, emi_52/1
  emi_52_bypass/1 -> cfblk133_out1bypassMux/2

== system gm_sampleModel71194_pp_7_1_sub/Subsystem/cfblk134_inst ==
  in1 : Inport  OutDataTypeStr=uint8  SampleTime=1
  in2 : Inport  Port=2  OutDataTypeStr=uint8  SampleTime=1
  mul_cfblk134_dotp_mulcomp : Product  Inputs=**  OutDataTypeStr=uint8  SampleTime=1
  out1 : Outport  OutDataTypeStr=uint8  SampleTime=1
  wires:
  in1/1 -> mul_cfblk134_dotp_mulcomp/1
  in2/1 -> mul_cfblk134_dotp_mulcomp/2
  mul_cfblk134_dotp_mulcomp/1 -> out1/1

== system gm_sampleModel71194_pp_7_1_sub/Subsystem/cfblk135 ==
  emi_59 : Inport  OutDataTypeStr=uint8  PortDimensions=1  SampleTime=1
  Action Port : Inport  Port=2  OutDataTypeStr=boolean  SampleTime=1
  cfblk135 : Gain  Gain="fi(0,0,8,7,\"hex\",\"80\")"  ParamDataTypeStr=fixdt(0, 8, 7)  OutDataTypeStr=fixdt(0, 16, 7)  SampleTime=1
  cfblk135_out1bypassMux : MultiPortSwitch  DataPortOrder=Zero-based contiguous  Inputs=2  zeroidx=on  OutDataTypeStr=fixdt(0, 16, 7)  SampleTime=1  SaturateOnIntegerOverflow=off  InputSameDT=off
  emi_60_bypass : UnitDelay  InitialCondition="fi(0,0,16,7,\"hex\",\"0000\")"  SampleTime=1
  emi_60 : Outport  SampleTime=1  InitialOutput=0
  wires:
  Action Port/1 -> cfblk135_out1bypassMux/1
  emi_59/1 -> cfblk135/1
  cfblk135/1 -> cfblk135_out1bypassMux/3
  cfblk135_out1bypassMux/1 -> emi_60_bypass/1, emi_60/1
  emi_60_bypass/1 -> cfblk135_out1bypassMux/2

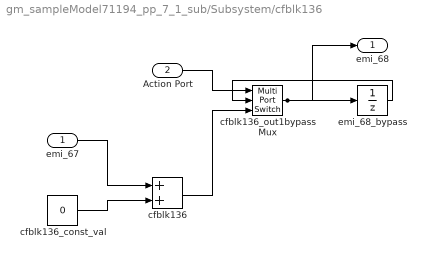
== system gm_sampleModel71194_pp_7_1_sub/Subsystem/cfblk136 ==
  emi_67 : Inport  OutDataTypeStr=uint8  PortDimensions=1  SampleTime=1
  Action Port : Inport  Port=2  OutDataTypeStr=boolean  SampleTime=1
  cfblk136 : Sum  OutDataTypeStr=uint8  AccumDataTypeStr=uint8  RndMeth=Nearest  SampleTime=1
  cfblk136_const_val : Constant  Value=0  VectorParams1D=off  OutDataTypeStr=uint8  SampleTime=1
  cfblk136_out1bypassMux : MultiPortSwitch  DataPortOrder=Zero-based contiguous  Inputs=2  zeroidx=on  OutDataTypeStr=uint8  SampleTime=1  SaturateOnIntegerOverflow=off  InputSameDT=off
  emi_68_bypass : UnitDelay  InitialCondition="fi(0,0,8,0,\"hex\",\"00\")"  SampleTime=1
  emi_68 : Outport  SampleTime=1  InitialOutput=0
  wires:
  Action Port/1 -> cfblk136_out1bypassMux/1
  emi_67/1 -> cfblk136/1
  cfblk136/1 -> cfblk136_out1bypassMux/3
  cfblk136_out1bypassMux/1 -> emi_68_bypass/1, emi_68/1
  emi_68_bypass/1 -> cfblk136_out1bypassMux/2
  cfblk136_const_val/1 -> cfblk136/2

== system gm_sampleModel71194_pp_7_1_sub/Subsystem/cfblk14 ==
  note: U(k)
  note: Edge
  U : Inport  OutDataTypeStr=uint8  SampleTime=1
  Delay Input1 : UnitDelay  Description=Store in Global RAM  DisableCoverage=on  InitialCondition=vinit  SampleTime=-1  HasFrameUpgradeWarning=on
  FixPt Relational Operator : RelationalOperator  Operator=>  OutDataTypeStr=fixdt(0, 8)  ZeroCross=off  InputSameDT=off
  Nonpositive : Subsystem  mask(Compare To Zero){relop=<=, OutDataTypeStr=boolean, ZeroCross=off}
      mask prompts: relop "Simulink:masks:Operator_MP"; OutDataTypeStr "Simulink:masks:OutputDataType_MP"; ZeroCross "Simulink:masks:EnableZerocrossingDetection_MP"
      mask help: Simulink:masks:CompareToZero_MD
      mask init:
      | OutDataTypeStr = 'boolean';
      | ZeroCross = 'off';
      | blkName = 'sampleModel71194_pp_7_1_sub/Subsystem/cfblk14/Nonpositive';
      | relop = '<=';
      | setValue = 'boolean';
      mask TypeOptions relop: == | ~= | < | <= | >= | >
      mask TypeOptions OutDataTypeStr: Simulink:masks:uint8 | Simulink:masks:boolean
      mask Callback ZeroCross: sl('zeroCrossEnable', gcbh);
      mask Display: disp([relop,' 0'])
  Y : Outport  SampleTime=1
  wires:
  U/1 -> Nonpositive/1(u)
  Delay Input1/1 -> FixPt Relational Operator/2
  FixPt Relational Operator/1 -> Y/1
  Nonpositive/1(y) -> FixPt Relational Operator/1, Delay Input1/1

== system gm_sampleModel71194_pp_7_1_sub/Subsystem/cfblk147 ==
  emi_83 : Inport  OutDataTypeStr=uint8  PortDimensions=1  SampleTime=1
  Action Port : Inport  Port=2  OutDataTypeStr=boolean  SampleTime=1
  cfblk147 : Signum  SampleTime=1
  cfblk147_out1bypassMux : MultiPortSwitch  DataPortOrder=Zero-based contiguous  Inputs=2  zeroidx=on  OutDataTypeStr=uint8  SampleTime=1  SaturateOnIntegerOverflow=off  InputSameDT=off
  emi_84_bypass : UnitDelay  InitialCondition="fi(0,0,8,0,\"hex\",\"00\")"  SampleTime=1
  emi_84 : Outport  SampleTime=1  InitialOutput=0
  wires:
  Action Port/1 -> cfblk147_out1bypassMux/1
  emi_83/1 -> cfblk147/1
  cfblk147/1 -> cfblk147_out1bypassMux/3
  cfblk147_out1bypassMux/1 -> emi_84_bypass/1, emi_84/1
  emi_84_bypass/1 -> cfblk147_out1bypassMux/2

== system gm_sampleModel71194_pp_7_1_sub/Subsystem/cfblk150 ==
  emi_91 : Inport  OutDataTypeStr=uint8  PortDimensions=1  SampleTime=1
  Action Port : Inport  Port=2  OutDataTypeStr=boolean  SampleTime=1
  cfblk150 : MinMax
  cfblk150_out1bypassMux : MultiPortSwitch  DataPortOrder=Zero-based contiguous  Inputs=2  zeroidx=on  OutDataTypeStr=uint8  SampleTime=1  SaturateOnIntegerOverflow=off  InputSameDT=off
  emi_92_bypass : UnitDelay  InitialCondition="fi(0,0,8,0,\"hex\",\"00\")"  SampleTime=1
  emi_92 : Outport  SampleTime=1  InitialOutput=0
  wires:
  Action Port/1 -> cfblk150_out1bypassMux/1
  emi_91/1 -> cfblk150/1
  cfblk150/1 -> cfblk150_out1bypassMux/3
  cfblk150_out1bypassMux/1 -> emi_92_bypass/1, emi_92/1
  emi_92_bypass/1 -> cfblk150_out1bypassMux/2

== system gm_sampleModel71194_pp_7_1_sub/Subsystem/cfblk153 ==
  emi_99 : Inport  OutDataTypeStr=uint8  PortDimensions=1  SampleTime=1
  Action Port : Inport  Port=2  OutDataTypeStr=boolean  SampleTime=1
  cfblk153 : Subsystem  mask(Real World Value Increment){}
      mask help: Simulink:masks:RealWorldValueIncrement_MD
      mask Display: disp('V++')
  cfblk153_out1bypassMux : MultiPortSwitch  DataPortOrder=Zero-based contiguous  Inputs=2  zeroidx=on  OutDataTypeStr=uint8  SampleTime=1  SaturateOnIntegerOverflow=off  InputSameDT=off
  emi_100_bypass : UnitDelay  InitialCondition="fi(0,0,8,0,\"hex\",\"00\")"  SampleTime=1
  emi_100 : Outport  SampleTime=1  InitialOutput=0
  wires:
  Action Port/1 -> cfblk153_out1bypassMux/1
  emi_99/1 -> cfblk153/1(u)
  cfblk153/1(y) -> cfblk153_out1bypassMux/3
  cfblk153_out1bypassMux/1 -> emi_100_bypass/1, emi_100/1
  emi_100_bypass/1 -> cfblk153_out1bypassMux/2

== system gm_sampleModel71194_pp_7_1_sub/Subsystem/cfblk160 ==
  In1 : Inport  OutDataTypeStr=uint8  PortDimensions=1  SampleTime=1
  Out1 : Outport  SampleTime=1  InitialOutput=[0]
  wires:
  In1/1 -> Out1/1

== system gm_sampleModel71194_pp_7_1_sub/Subsystem/cfblk161 ==
  In1 : Inport  OutDataTypeStr=uint8  PortDimensions=1  SampleTime=1
  Out1 : Outport  SampleTime=1  InitialOutput=[0]
  wires:
  In1/1 -> Out1/1

== system gm_sampleModel71194_pp_7_1_sub/Subsystem/cfblk162 ==
  In1 : Inport  OutDataTypeStr=uint8  PortDimensions=1  SampleTime=1
  Out1 : Outport  SampleTime=1  InitialOutput=[0]
  wires:
  In1/1 -> Out1/1

== system gm_sampleModel71194_pp_7_1_sub/Subsystem/cfblk17 ==
  emi_107 : Inport  OutDataTypeStr=uint8  PortDimensions=1  SampleTime=1
  Action Port : Inport  Port=2  OutDataTypeStr=boolean  SampleTime=1
  cfblk17 : MinMax
  cfblk17_out1bypassMux : MultiPortSwitch  DataPortOrder=Zero-based contiguous  Inputs=2  zeroidx=on  OutDataTypeStr=uint8  SampleTime=1  SaturateOnIntegerOverflow=off  InputSameDT=off
  emi_108_bypass : UnitDelay  InitialCondition="fi(0,0,8,0,\"hex\",\"00\")"  SampleTime=1
  emi_108 : Outport  SampleTime=1  InitialOutput=0
  wires:
  Action Port/1 -> cfblk17_out1bypassMux/1
  emi_107/1 -> cfblk17/1
  cfblk17/1 -> cfblk17_out1bypassMux/3
  cfblk17_out1bypassMux/1 -> emi_108_bypass/1, emi_108/1
  emi_108_bypass/1 -> cfblk17_out1bypassMux/2

== system gm_sampleModel71194_pp_7_1_sub/Subsystem/cfblk174 ==
  emi_75 : Inport  OutDataTypeStr=uint8  PortDimensions=1  SampleTime=1
  Action Port : Inport  Port=2  OutDataTypeStr=boolean  SampleTime=1
  cfblk174 : Subsystem
      settings: MinAlgLoopOccurrences=on
  emi_76 : Outport  SampleTime=1  InitialOutput=0
  wires:
  Action Port/1 -> cfblk174/Enable
  emi_75/1 -> cfblk174/1(in0)
  cfblk174/1(out0) -> emi_76/1

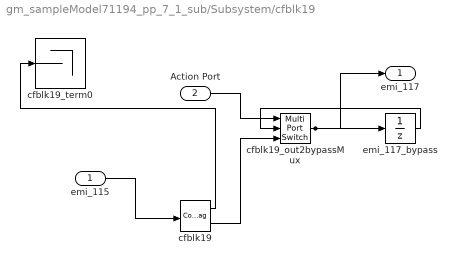
== system gm_sampleModel71194_pp_7_1_sub/Subsystem/cfblk19 ==
  emi_115 : Inport  OutDataTypeStr=uint8  PortDimensions=1  SampleTime=1
  Action Port : Inport  Port=2  OutDataTypeStr=boolean  SampleTime=1
  cfblk19 : ComplexToRealImag  SampleTime=1
  cfblk19_out2bypassMux : MultiPortSwitch  DataPortOrder=Zero-based contiguous  Inputs=2  zeroidx=on  OutDataTypeStr=uint8  SampleTime=1  SaturateOnIntegerOverflow=off  InputSameDT=off
  cfblk19_term0 : Terminator
  emi_117_bypass : UnitDelay  InitialCondition="fi(0,0,8,0,\"hex\",\"00\")"  SampleTime=1
  emi_117 : Outport  SampleTime=1  InitialOutput=0
  wires:
  Action Port/1 -> cfblk19_out2bypassMux/1
  emi_115/1 -> cfblk19/1
  cfblk19/1 -> cfblk19_term0/1
  cfblk19/2 -> cfblk19_out2bypassMux/3
  cfblk19_out2bypassMux/1 -> emi_117_bypass/1, emi_117/1
  emi_117_bypass/1 -> cfblk19_out2bypassMux/2

== system gm_sampleModel71194_pp_7_1_sub/Subsystem/cfblk2 ==
  emi_124 : Inport  OutDataTypeStr=uint8  PortDimensions=1  SampleTime=1
  Action Port : Inport  Port=2  OutDataTypeStr=boolean  SampleTime=1
  cfblk2 : Subsystem  mask(Compare To Constant){relop=<=, const=double(3), OutDataTypeStr=uint8, ZeroCross=on}
      mask prompts: relop "Simulink:masks:Operator_MP"; const "Simulink:masks:ConstantValue_MP"; OutDataTypeStr "Simulink:masks:OutputDataType_MP"; ZeroCross "Simulink:masks:EnableZerocrossingDetection_MP"
      mask help: Simulink:masks:CompareToConstant_MD
      mask init:
      | OutDataTypeStr = 'uint8';
      | ZeroCross = 'on';
      | blkName = 'sampleModel71194_pp_7_1_sub/Subsystem/cfblk2/cfblk2';
      | const = double(3);
      | const_str = '3.0';
      | const_val = double(3);
      | relop = '<=';
      | setValue = 'fixdt(0, 8)';
      | str = '<= 3';
      mask TypeOptions relop: == | ~= | < | <= | >= | >
      mask TypeOptions OutDataTypeStr: Simulink:masks:uint8 | Simulink:masks:boolean
      mask Callback ZeroCross: sl('zeroCrossEnable', gcbh);
      mask Display: disp(str)
  cfblk2_out1bypassMux : MultiPortSwitch  DataPortOrder=Zero-based contiguous  Inputs=2  zeroidx=on  OutDataTypeStr=uint8  SampleTime=1  SaturateOnIntegerOverflow=off  InputSameDT=off
  emi_125_bypass : UnitDelay  InitialCondition="fi(0,0,8,0,\"hex\",\"00\")"  SampleTime=1
  emi_125 : Outport  SampleTime=1  InitialOutput=0
  wires:
  Action Port/1 -> cfblk2_out1bypassMux/1
  emi_124/1 -> cfblk2/1(u)
  cfblk2/1(y) -> cfblk2_out1bypassMux/3
  cfblk2_out1bypassMux/1 -> emi_125_bypass/1, emi_125/1
  emi_125_bypass/1 -> cfblk2_out1bypassMux/2

== system gm_sampleModel71194_pp_7_1_sub/Subsystem/cfblk204 ==
  emi_132 : Inport  OutDataTypeStr=uint8  PortDimensions=1  SampleTime=1
  Action Port : Inport  Port=2  OutDataTypeStr=boolean  SampleTime=1
  cfblk204 : DataTypeConversion  OutDataTypeStr=fixdt(0,8,0)
  cfblk204_out1bypassMux : MultiPortSwitch  DataPortOrder=Zero-based contiguous  Inputs=2  zeroidx=on  OutDataTypeStr=uint8  SampleTime=1  SaturateOnIntegerOverflow=off  InputSameDT=off
  emi_133_bypass : UnitDelay  InitialCondition="fi(0,0,8,0,\"hex\",\"00\")"  SampleTime=1
  emi_133 : Outport  SampleTime=1  InitialOutput=0
  wires:
  Action Port/1 -> cfblk204_out1bypassMux/1
  emi_132/1 -> cfblk204/1
  cfblk204/1 -> cfblk204_out1bypassMux/3
  cfblk204_out1bypassMux/1 -> emi_133_bypass/1, emi_133/1
  emi_133_bypass/1 -> cfblk204_out1bypassMux/2

== system gm_sampleModel71194_pp_7_1_sub/Subsystem/cfblk206 ==
  emi_140 : Inport  OutDataTypeStr=uint8  PortDimensions=1  SampleTime=1
  Action Port : Inport  Port=2  OutDataTypeStr=boolean  SampleTime=1
  cfblk206 : DataTypeConversion  OutDataTypeStr=fixdt(0,8,0)
  cfblk206_out1bypassMux : MultiPortSwitch  DataPortOrder=Zero-based contiguous  Inputs=2  zeroidx=on  OutDataTypeStr=uint8  SampleTime=1  SaturateOnIntegerOverflow=off  InputSameDT=off
  emi_141_bypass : UnitDelay  InitialCondition="fi(0,0,8,0,\"hex\",\"00\")"  SampleTime=1
  emi_141 : Outport  SampleTime=1  InitialOutput=0
  wires:
  Action Port/1 -> cfblk206_out1bypassMux/1
  emi_140/1 -> cfblk206/1
  cfblk206/1 -> cfblk206_out1bypassMux/3
  cfblk206_out1bypassMux/1 -> emi_141_bypass/1, emi_141/1
  emi_141_bypass/1 -> cfblk206_out1bypassMux/2

== system gm_sampleModel71194_pp_7_1_sub/Subsystem/cfblk209 ==
  emi_148 : Inport  OutDataTypeStr=uint8  PortDimensions=1  SampleTime=1
  Action Port : Inport  Port=2  OutDataTypeStr=boolean  SampleTime=1
  cfblk209 : DataTypeConversion  OutDataTypeStr=boolean  SampleTime=1  SaturateOnIntegerOverflow=off  RndMeth=Floor
  cfblk209_out1bypassMux : MultiPortSwitch  DataPortOrder=Zero-based contiguous  Inputs=2  zeroidx=on  SampleTime=1  SaturateOnIntegerOverflow=off  InputSameDT=off
  emi_149_bypass : UnitDelay  SampleTime=1
  emi_149 : Outport  SampleTime=1  InitialOutput=0
  wires:
  Action Port/1 -> cfblk209_out1bypassMux/1
  emi_148/1 -> cfblk209/1
  cfblk209/1 -> cfblk209_out1bypassMux/3
  cfblk209_out1bypassMux/1 -> emi_149_bypass/1, emi_149/1
  emi_149_bypass/1 -> cfblk209_out1bypassMux/2

== system gm_sampleModel71194_pp_7_1_sub/Subsystem/cfblk211 ==
  emi_156 : Inport  OutDataTypeStr=uint8  PortDimensions=1  SampleTime=1
  Action Port : Inport  Port=2  OutDataTypeStr=boolean  SampleTime=1
  cfblk211 : DataTypeConversion  OutDataTypeStr=boolean  SampleTime=1  SaturateOnIntegerOverflow=off  RndMeth=Floor
  cfblk211_out1bypassMux : MultiPortSwitch  DataPortOrder=Zero-based contiguous  Inputs=2  zeroidx=on  SampleTime=1  SaturateOnIntegerOverflow=off  InputSameDT=off
  emi_157_bypass : UnitDelay  SampleTime=1
  emi_157 : Outport  SampleTime=1  InitialOutput=0
  wires:
  Action Port/1 -> cfblk211_out1bypassMux/1
  emi_156/1 -> cfblk211/1
  cfblk211/1 -> cfblk211_out1bypassMux/3
  cfblk211_out1bypassMux/1 -> emi_157_bypass/1, emi_157/1
  emi_157_bypass/1 -> cfblk211_out1bypassMux/2

== system gm_sampleModel71194_pp_7_1_sub/Subsystem/cfblk213 ==
  emi_172 : Inport  OutDataTypeStr=uint8  PortDimensions=1  SampleTime=1
  Action Port : Inport  Port=2  OutDataTypeStr=boolean  SampleTime=1
  cfblk213 : DataTypeConversion  OutDataTypeStr=boolean  SampleTime=1  SaturateOnIntegerOverflow=off  RndMeth=Floor
  cfblk213_out1bypassMux : MultiPortSwitch  DataPortOrder=Zero-based contiguous  Inputs=2  zeroidx=on  SampleTime=1  SaturateOnIntegerOverflow=off  InputSameDT=off
  emi_173_bypass : UnitDelay  SampleTime=1
  emi_173 : Outport  SampleTime=1  InitialOutput=0
  wires:
  Action Port/1 -> cfblk213_out1bypassMux/1
  emi_172/1 -> cfblk213/1
  cfblk213/1 -> cfblk213_out1bypassMux/3
  cfblk213_out1bypassMux/1 -> emi_173_bypass/1, emi_173/1
  emi_173_bypass/1 -> cfblk213_out1bypassMux/2
